simulink model "PWR"  (R2019b)
settings: Solver=VariableStepAuto  StartTime=0.0  StopTime=10.0  RelTol=1e-3
settings Model: Creator=YJR  LastModifiedBy=YJR

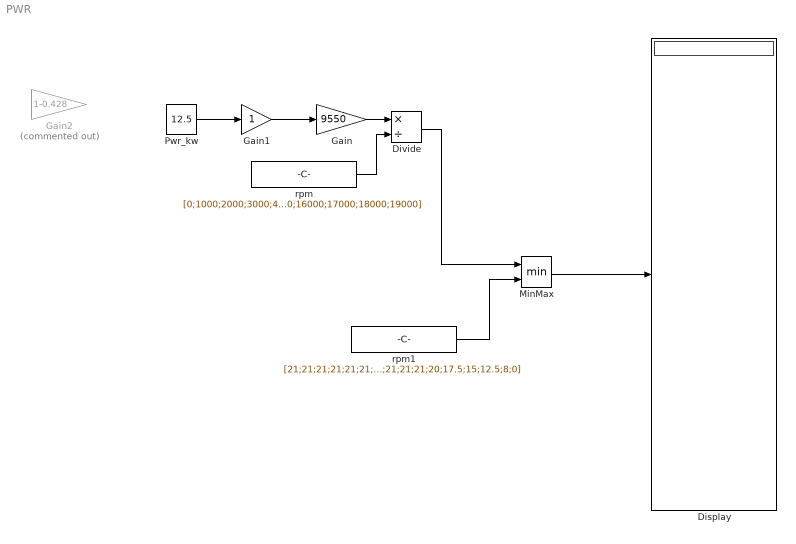
== system PWR ==
  Display : Display
  Divide : Product  Inputs=*/
  Gain : Gain  Gain=9550
  Gain1 : Gain
  Gain2 : Gain  Commented=on  Gain=1-0.428
  MinMax : MinMax  Inputs=2
  Pwr_kw : Constant  Value=12.5
  rpm : Constant  Value=[0;1000;2000;3000;4000;5000;6000;7000;8000;9000;10000;11000;12000;13000;14000;15000;16000;17000;18000;19000]
  rpm1 : Constant  Value=[21;21;21;21;21;21;21;21;21;21;21;21;21;21;20;17.5;15;12.5;8;0]
  wires:
  Gain/1 -> Divide/1
  rpm/1 -> Divide/2
  Divide/1 -> MinMax/1
  MinMax/1 -> Display/1
  rpm1/1 -> MinMax/2
  Pwr_kw/1 -> Gain1/1
  Gain1/1 -> Gain/1
